simulink model "equivalent"  (R2018a)
settings: Solver=VariableStepAuto  StartTime=0.0  StopTime=10.0  RelTol=1e-3
undefined symbols (not defined in the file): DiscIntNeverNeededParam, sigbuilder_block
libraries: simulink x479
(part 2 of 10)

== system equivalent/cfblk286 ==
  cfblk1 : Inport
  Action Port : ActionPort  ActionType=else
  cfblk11 : Subsystem  TreatAsAtomicUnit=on
  cfblk12 : Subsystem  TreatAsAtomicUnit=on
  cfblk13 : Delay
  cfblk14 : Delay
  cfblk15 : Delay
  cfblk3 : DiscreteFir
  cfblk4 : simulink/Discrete/Transfer Fcn Real Zero  ZeroZ=0.75  ICPrevInput=0.0  DoSatur=off
      settings: SourceProductName=Simulink  SourceProductBaseCode=SL
  cfblk5 : DiscreteZeroPole  Poles=[0 0.5]  Gain=1  SampleTime=-1
  cfblk6 : simulink/Discrete/Difference  ICPrevInput=0.0  OutMin=[]  OutMax=[]  OutDataTypeStr=Inherit: Inherit via back propagation  OutDataType=fixdt(1, 16)  OutScaling=2^-10  DoSatur=off
  cfblk7 : Delay  ShowEnablePort=on
      settings: InputPortMap=u0,e6
  cfblk8 : DiscreteFir
  cfblk9 : If  SampleTime=1
  cyemi_{125,134..136,154..164} (15 alike) : DataTypeConversion  OutDataTypeStr=double
  cfblk2 : Outport
  cfblk10 : Outport  Port=2
  wires:
  cfblk6/1 -> cfblk2/1
  cfblk8/1 -> cyemi_155/1, cyemi_156/1
  cfblk5/1 -> cyemi_154/1, cyemi_160/1
  cfblk11/2(cfblk9) -> cfblk10/1
  cfblk12/1(cfblk2) -> cyemi_125/1, cyemi_162/1, cyemi_163/1
  cfblk9/1 -> cfblk11/Action
  cfblk9/2 -> cfblk12/Action
  cyemi_125/1 -> cfblk11/1(cfblk1)
  cyemi_134/1 -> cfblk12/1(cfblk1)
  cfblk1/1 -> cyemi_134/1
  cyemi_135/1 -> cfblk12/2(cfblk16)
  cfblk13/1 -> cyemi_135/1
  cyemi_136/1 -> cfblk12/3(cfblk17)
  cfblk15/1 -> cyemi_136/1
  cyemi_154/1 -> cfblk13/1
  cyemi_155/1 -> cfblk14/1
  cyemi_156/1 -> cfblk15/1
  cyemi_157/1 -> cfblk3/1
  cfblk7/1 -> cyemi_157/1
  cyemi_158/1 -> cfblk4/1
  cfblk11/1(cfblk2) -> cyemi_158/1
  cyemi_159/1 -> cfblk5/1
  cfblk3/1 -> cyemi_159/1
  cyemi_160/1 -> cfblk6/1
  cyemi_161/1 -> cfblk7/1
  cfblk4/1 -> cyemi_161/1
  cyemi_162/1 -> cfblk7/2
  cyemi_163/1 -> cfblk8/1
  cyemi_164/1 -> cfblk9/1
  cfblk14/1 -> cyemi_164/1

== system equivalent/cfblk287 ==
  cfblk1 : Inport
  cfblk12 : Inport  Port=2
  Action Port : ActionPort  ActionType=then
  cfblk10 : DiscreteTransferFcn
  cfblk11 : If  SampleTime=1
  cfblk15 : Subsystem  TreatAsAtomicUnit=on
  cfblk16 : Subsystem  TreatAsAtomicUnit=on
  cfblk{9,17..19} (4 alike) : Delay
  cfblk3 : Delay  DelayLengthSource=Input port
      settings: InputPortMap=u0,p1
  cfblk4 : simulink/Discrete/Transfer Fcn First Order  PoleZ=0.95  ICPrevOutput=0.0  DoSatur=off
      settings: SourceProductName=Simulink
  cfblk5 : DiscreteIntegrator  SampleTime=-1  ICPrevOutput=DiscIntNeverNeededParam  ICPrevScaledInput=DiscIntNeverNeededParam
  cfblk6 : simulink/Discrete/Transfer Fcn Real Zero  ZeroZ=0.75  ICPrevInput=0.0  DoSatur=off
      settings: SourceProductName=Simulink  SourceProductBaseCode=SL
  cfblk7 : Delay  ShowEnablePort=on
      settings: InputPortMap=u0,e6
  cfblk8 : simulink/Discrete/Transfer Fcn Real Zero  ZeroZ=0.75  ICPrevInput=0.0  DoSatur=off
      settings: SourceProductName=Simulink  SourceProductBaseCode=SL
  cyemi_{167..169,179..180,190..201} (17 alike) : DataTypeConversion  OutDataTypeStr=double
  cfblk2 : Outport
  cfblk13 : Outport  Port=2
  cfblk14 : Outport  Port=3
  wires:
  cfblk4/1 -> cfblk2/1
  cfblk7/1 -> cfblk14/1, cyemi_180/1
  cfblk15/3(cfblk12) -> cfblk13/1
  cfblk10/1 -> cyemi_179/1, cyemi_194/1
  cfblk11/1 -> cfblk15/Action
  cfblk11/2 -> cfblk16/Action
  cyemi_167/1 -> cfblk10/1
  cfblk1/1 -> cyemi_167/1
  cyemi_168/1 -> cfblk11/1
  cfblk19/1 -> cyemi_168/1
  cyemi_169/1 -> cfblk15/1(cfblk1)
  cfblk17/1 -> cyemi_169/1
  cyemi_179/1 -> cfblk16/1(cfblk1)
  cyemi_180/1 -> cfblk16/2(cfblk12)
  cyemi_190/1 -> cfblk17/1
  cfblk8/1 -> cyemi_190/1
  cyemi_191/1 -> cfblk18/1
  cfblk15/2(cfblk11) -> cyemi_191/1
  cyemi_192/1 -> cfblk19/1
  cfblk6/1 -> cyemi_192/1
  cyemi_193/1 -> cfblk3/1
  cfblk18/1 -> cyemi_193/1
  cyemi_194/1 -> cfblk3/2
  cyemi_195/1 -> cfblk4/1
  cfblk15/1(cfblk2) -> cyemi_195/1
  cyemi_196/1 -> cfblk5/1
  cfblk12/1 -> cyemi_196/1
  cyemi_197/1 -> cfblk6/1
  cfblk9/1 -> cyemi_197/1
  cyemi_198/1 -> cfblk7/1
  cfblk3/1 -> cyemi_198/1
  cyemi_199/1 -> cfblk7/2
  cfblk5/1 -> cyemi_199/1
  cyemi_200/1 -> cfblk8/1
  cfblk16/1(cfblk2) -> cyemi_200/1
  cyemi_201/1 -> cfblk9/1
  cfblk16/2(cfblk13) -> cyemi_201/1

== system equivalent/cfblk288 ==
  cfblk1 : Inport
  cfblk7 : Inport  Port=2
  Action Port : ActionPort  ActionType=else
  cfblk3 : DiscreteStateSpace  SampleTime=-1
  cfblk4 : simulink/Discrete/Transfer Fcn Real Zero  ZeroZ=0.75  ICPrevInput=0.0  DoSatur=off
      settings: SourceProductName=Simulink  SourceProductBaseCode=SL
  cfblk5 : simulink/Continuous/PID Controller (2DOF)  Controller=PID  TimeDomain=Discrete-time  SampleTime=-1  IntegratorMethod=Forward Euler  FilterMethod=Forward Euler  Form=Parallel  UseFilter=on  ControllerParametersSource=internal  P=1  I=1  D=0  N=100  b=1  c=1  InitialConditionSource=internal  InitialConditionForIntegrator=0  InitialConditionForFilter=0  ExternalReset=none  LimitOutput=off  UpperSaturationLimit=inf  LowerSaturationLimit=-inf  LinearizeAsGain=off  AntiWindupMode=none  Kb=1  TrackingMode=off  Kt=1  PParamMin=[]  PParamMax=[]  IParamMin=[]  IParamMax=[]  DParamMin=[]  DParamMax=[]  NParamMin=[]  NParamMax=[]  bParamMin=[]  bParamMax=[]  cParamMin=[]  cParamMax=[]  KbParamMin=[]  KbParamMax=[]  KtParamMin=[]  KtParamMax=[]  POutMin=[]  POutMax=[]  IOutMin=[]  IOutMax=[]  DOutMin=[]  DOutMax=[]  NOutMin=[]  NOutMax=[]  bOutMin=[]  bOutMax=[]  cOutMin=[]  cOutMax=[]  KbOutMin=[]  KbOutMax=[]  KtOutMin=[]  KtOutMax=[]  IntegratorOutMin=[]  IntegratorOutMax=[]  FilterOutMin=[]  FilterOutMax=[]  SumOutMin=[]  SumOutMax=[]  Sum1OutMin=[]  Sum1OutMax=[]  Sum2OutMin=[]  Sum2OutMax=[]  Sum3OutMin=[]  Sum3OutMax=[]  SumI1OutMin=[]  SumI1OutMax=[]  SumI2OutMin=[]  SumI2OutMax=[]  SumI3OutMin=[]  SumI3OutMax=[]  SumDOutMin=[]  SumDOutMax=[]  SaturationOutMin=[]  SaturationOutMax=[]  IntegratorContinuousStateAttributes=''  IntegratorStateMustResolveToSignalObject=off  IntegratorRTWStateStorageClass=Auto  FilterContinuousStateAttributes=''  FilterStateMustResolveToSignalObject=off  FilterRTWStateStorageClass=Auto  DifferentiatorICPrevScaledInput=0  DifferentiatorOutMin=[]  DifferentiatorOutMax=[]  FilterDiffOutCoefMin=[]  FilterDiffOutCoefMax=[]  SumDenOutMin=[]  SumDenOutMax=[]  SumNumOutMin=[]  SumNumOutMax=[]  ReciprocalOutMin=[]  ReciprocalOutMax=[]  DivideOutMin=[]  DivideOutMax=[]  TunerSelectOption=Transfer Function Based (PID Tuner App)
  cfblk6 : Delay  ShowEnablePort=on
      settings: InputPortMap=u0,e6
  cyemi_{204..209} (6 alike) : DataTypeConversion  OutDataTypeStr=double
  cfblk2 : Outport
  cfblk8 : Outport  Port=2
  cfblk9 : Outport  Port=3
  wires:
  cfblk6/1 -> cfblk2/1
  cfblk3/1 -> cfblk8/1, cyemi_206/1
  cfblk7/1 -> cfblk9/1, cyemi_205/1, cyemi_207/1
  cyemi_204/1 -> cfblk3/1
  cfblk1/1 -> cyemi_204/1
  cyemi_205/1 -> cfblk4/1
  cyemi_206/1 -> cfblk5/1
  cyemi_207/1 -> cfblk5/2
  cyemi_208/1 -> cfblk6/1
  cfblk5/1 -> cyemi_208/1
  cyemi_209/1 -> cfblk6/2
  cfblk4/1 -> cyemi_209/1

== system equivalent/cfblk289 ==
  cfblk1 : Inport
  cfblk6 : Inport  Port=2
  Action Port : ActionPort  ActionType=then
  cfblk3 : DiscreteZeroPole  Poles=[0 0.5]  Gain=1  SampleTime=-1
  cfblk4 : DiscreteFilter
  cfblk5 : DiscreteStateSpace  SampleTime=-1
  cyemi_212 : DataTypeConversion  OutDataTypeStr=double
  cyemi_213 : DataTypeConversion  OutDataTypeStr=double
  cyemi_214 : DataTypeConversion  OutDataTypeStr=double
  cfblk2 : Outport
  cfblk7 : Outport  Port=2
  wires:
  cfblk4/1 -> cfblk2/1
  cfblk1/1 -> cfblk7/1
  cyemi_212/1 -> cfblk3/1
  cfblk5/1 -> cyemi_212/1
  cyemi_213/1 -> cfblk4/1
  cfblk3/1 -> cyemi_213/1
  cyemi_214/1 -> cfblk5/1
  cfblk6/1 -> cyemi_214/1

== system equivalent/cfblk290 ==
  cfblk1 : Inport
  cfblk9 : Inport  Port=2
  cfblk10 : Inport  Port=3
  Action Port : ActionPort  ActionType=else
  cfblk12 : Delay
  cfblk3 : DiscreteZeroPole  Poles=[0 0.5]  Gain=1  SampleTime=-1
  cfblk4 : simulink/Discrete/Tapped Delay  vinit=0.0  samptime=-1  NumDelays=1  DelayOrder=Oldest  includeCurrent=off
  cfblk5 : Delay  ShowEnablePort=on
      settings: InputPortMap=u0,e6
  cfblk6 : simulink/Continuous/PID Controller (2DOF)  Controller=PID  TimeDomain=Discrete-time  SampleTime=-1  IntegratorMethod=Forward Euler  FilterMethod=Forward Euler  Form=Parallel  UseFilter=on  ControllerParametersSource=internal  P=1  I=1  D=0  N=100  b=1  c=1  InitialConditionSource=internal  InitialConditionForIntegrator=0  InitialConditionForFilter=0  ExternalReset=none  LimitOutput=off  UpperSaturationLimit=inf  LowerSaturationLimit=-inf  LinearizeAsGain=off  AntiWindupMode=none  Kb=1  TrackingMode=off  Kt=1  PParamMin=[]  PParamMax=[]  IParamMin=[]  IParamMax=[]  DParamMin=[]  DParamMax=[]  NParamMin=[]  NParamMax=[]  bParamMin=[]  bParamMax=[]  cParamMin=[]  cParamMax=[]  KbParamMin=[]  KbParamMax=[]  KtParamMin=[]  KtParamMax=[]  POutMin=[]  POutMax=[]  IOutMin=[]  IOutMax=[]  DOutMin=[]  DOutMax=[]  NOutMin=[]  NOutMax=[]  bOutMin=[]  bOutMax=[]  cOutMin=[]  cOutMax=[]  KbOutMin=[]  KbOutMax=[]  KtOutMin=[]  KtOutMax=[]  IntegratorOutMin=[]  IntegratorOutMax=[]  FilterOutMin=[]  FilterOutMax=[]  SumOutMin=[]  SumOutMax=[]  Sum1OutMin=[]  Sum1OutMax=[]  Sum2OutMin=[]  Sum2OutMax=[]  Sum3OutMin=[]  Sum3OutMax=[]  SumI1OutMin=[]  SumI1OutMax=[]  SumI2OutMin=[]  SumI2OutMax=[]  SumI3OutMin=[]  SumI3OutMax=[]  SumDOutMin=[]  SumDOutMax=[]  SaturationOutMin=[]  SaturationOutMax=[]  IntegratorContinuousStateAttributes=''  IntegratorStateMustResolveToSignalObject=off  IntegratorRTWStateStorageClass=Auto  FilterContinuousStateAttributes=''  FilterStateMustResolveToSignalObject=off  FilterRTWStateStorageClass=Auto  DifferentiatorICPrevScaledInput=0  DifferentiatorOutMin=[]  DifferentiatorOutMax=[]  FilterDiffOutCoefMin=[]  FilterDiffOutCoefMax=[]  SumDenOutMin=[]  SumDenOutMax=[]  SumNumOutMin=[]  SumNumOutMax=[]  ReciprocalOutMin=[]  ReciprocalOutMax=[]  DivideOutMin=[]  DivideOutMax=[]  TunerSelectOption=Transfer Function Based (PID Tuner App)
  cfblk7 : simulink/Discrete/Difference  ICPrevInput=0.0  OutMin=[]  OutMax=[]  OutDataTypeStr=Inherit: Inherit via back propagation  OutDataType=fixdt(1, 16)  OutScaling=2^-10  DoSatur=off
  cfblk8 : DiscreteIntegrator  SampleTime=-1  ICPrevOutput=DiscIntNeverNeededParam  ICPrevScaledInput=DiscIntNeverNeededParam
  cyemi_{219..227} (9 alike) : DataTypeConversion  OutDataTypeStr=double
  cfblk2 : Outport
  cfblk11 : Outport  Port=2
  wires:
  cfblk10/1 -> cyemi_223/1, cyemi_225/1
  cfblk6/1 -> cfblk11/1
  cfblk9/1 -> cfblk2/1
  cyemi_219/1 -> cfblk12/1
  cfblk5/1 -> cyemi_219/1
  cyemi_220/1 -> cfblk3/1
  cfblk12/1 -> cyemi_220/1
  cyemi_221/1 -> cfblk4/1
  cfblk8/1 -> cyemi_221/1
  cyemi_222/1 -> cfblk5/1
  cfblk3/1 -> cyemi_222/1
  cyemi_223/1 -> cfblk5/2
  cyemi_224/1 -> cfblk6/1
  cfblk7/1 -> cyemi_224/1
  cyemi_225/1 -> cfblk6/2
  cyemi_226/1 -> cfblk7/1
  cfblk4/1 -> cyemi_226/1
  cyemi_227/1 -> cfblk8/1
  cfblk1/1 -> cyemi_227/1

== system equivalent/cfblk291 ==
  cfblk1 : Inport
  cfblk7 : Inport  Port=2
  Action Port : ActionPort  ActionType=then
  cfblk3 : simulink/Discrete/Tapped Delay  vinit=0.0  samptime=-1  NumDelays=1  DelayOrder=Oldest  includeCurrent=off
  cfblk4 : simulink/Continuous/PID Controller  Controller=PID  TimeDomain=Discrete-time  SampleTime=-1  IntegratorMethod=Forward Euler  FilterMethod=Forward Euler  Form=Parallel  UseFilter=on  ControllerParametersSource=internal  P=1  I=1  D=0  N=100  InitialConditionSource=internal  InitialConditionForIntegrator=0  InitialConditionForFilter=0  ExternalReset=none  LimitOutput=off  UpperSaturationLimit=inf  LowerSaturationLimit=-inf  LinearizeAsGain=off  AntiWindupMode=none  Kb=1  TrackingMode=off  Kt=1  PParamMin=[]  PParamMax=[]  IParamMin=[]  IParamMax=[]  DParamMin=[]  DParamMax=[]  NParamMin=[]  NParamMax=[]  KbParamMin=[]  KbParamMax=[]  KtParamMin=[]  KtParamMax=[]  POutMin=[]  POutMax=[]  IOutMin=[]  IOutMax=[]  DOutMin=[]  DOutMax=[]  NOutMin=[]  NOutMax=[]  KbOutMin=[]  KbOutMax=[]  KtOutMin=[]  KtOutMax=[]  IntegratorOutMin=[]  IntegratorOutMax=[]  FilterOutMin=[]  FilterOutMax=[]  SumOutMin=[]  SumOutMax=[]  SumI1OutMin=[]  SumI1OutMax=[]  SumI2OutMin=[]  SumI2OutMax=[]  SumI3OutMin=[]  SumI3OutMax=[]  SumDOutMin=[]  SumDOutMax=[]  SaturationOutMin=[]  SaturationOutMax=[]  IntegratorContinuousStateAttributes=''  IntegratorStateMustResolveToSignalObject=off  IntegratorRTWStateStorageClass=Auto  FilterContinuousStateAttributes=''  FilterStateMustResolveToSignalObject=off  FilterRTWStateStorageClass=Auto  DifferentiatorICPrevScaledInput=0  DifferentiatorOutMin=[]  DifferentiatorOutMax=[]  FilterDiffOutCoefMin=[]  FilterDiffOutCoefMax=[]  SumDenOutMin=[]  SumDenOutMax=[]  SumNumOutMin=[]  SumNumOutMax=[]  ReciprocalOutMin=[]  ReciprocalOutMax=[]  DivideOutMin=[]  DivideOutMax=[]  TunerSelectOption=Transfer Function Based (PID Tuner App)
  cfblk5 : DiscreteFilter
  cfblk6 : UnitDelay  SampleTime=-1
  cyemi_{230..233} (4 alike) : DataTypeConversion  OutDataTypeStr=double
  cfblk2 : Outport
  cfblk8 : Outport  Port=2
  cfblk9 : Outport  Port=3
  wires:
  cfblk5/1 -> cfblk2/1
  cfblk4/1 -> cfblk8/1
  cfblk3/1 -> cfblk9/1
  cfblk1/1 -> cyemi_232/1, cyemi_233/1
  cyemi_230/1 -> cfblk3/1
  cfblk7/1 -> cyemi_230/1
  cyemi_231/1 -> cfblk4/1
  cfblk6/1 -> cyemi_231/1
  cyemi_232/1 -> cfblk5/1
  cyemi_233/1 -> cfblk6/1

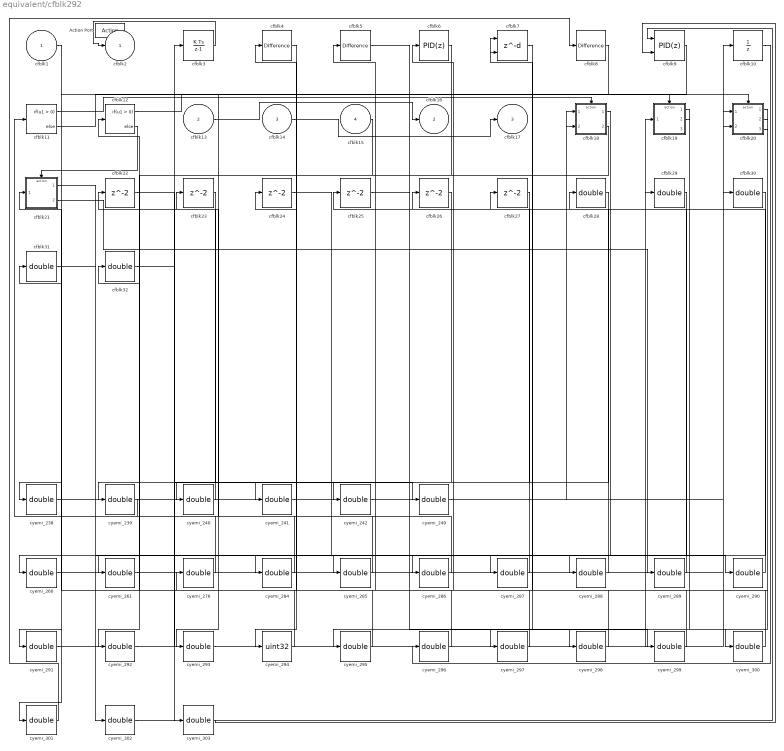
== system equivalent/cfblk292 ==
  cfblk1 : Inport
  cfblk13 : Inport  Port=2
  cfblk14 : Inport  Port=3
  cfblk15 : Inport  Port=4
  Action Port : ActionPort  ActionType=else
  cfblk10 : UnitDelay  SampleTime=-1
  cfblk11 : If  SampleTime=1
  cfblk12 : If  SampleTime=1
  cfblk18 : Subsystem  TreatAsAtomicUnit=on
  cfblk19 : Subsystem  TreatAsAtomicUnit=on
  cfblk20 : Subsystem  TreatAsAtomicUnit=on
  cfblk21 : Subsystem  TreatAsAtomicUnit=on
  cfblk{22..27} (6 alike) : Delay
  cfblk{28..32} (5 alike) : DataTypeConversion  OutDataTypeStr=double
  cfblk3 : DiscreteIntegrator  SampleTime=-1  ICPrevOutput=DiscIntNeverNeededParam  ICPrevScaledInput=DiscIntNeverNeededParam
  cfblk4 : simulink/Discrete/Difference  ICPrevInput=0.0  OutMin=[]  OutMax=[]  OutDataTypeStr=Inherit: Inherit via back propagation  OutDataType=fixdt(1, 16)  OutScaling=2^-10  DoSatur=off
  cfblk5 : simulink/Discrete/Difference  ICPrevInput=0.0  OutMin=[]  OutMax=[]  OutDataTypeStr=Inherit: Inherit via back propagation  OutDataType=fixdt(1, 16)  OutScaling=2^-10  DoSatur=off
  cfblk6 : simulink/Continuous/PID Controller  Controller=PID  TimeDomain=Discrete-time  SampleTime=-1  IntegratorMethod=Forward Euler  FilterMethod=Forward Euler  Form=Parallel  UseFilter=on  ControllerParametersSource=internal  P=1  I=1  D=0  N=100  InitialConditionSource=internal  InitialConditionForIntegrator=0  InitialConditionForFilter=0  ExternalReset=none  LimitOutput=off  UpperSaturationLimit=inf  LowerSaturationLimit=-inf  LinearizeAsGain=off  AntiWindupMode=none  Kb=1  TrackingMode=off  Kt=1  PParamMin=[]  PParamMax=[]  IParamMin=[]  IParamMax=[]  DParamMin=[]  DParamMax=[]  NParamMin=[]  NParamMax=[]  KbParamMin=[]  KbParamMax=[]  KtParamMin=[]  KtParamMax=[]  POutMin=[]  POutMax=[]  IOutMin=[]  IOutMax=[]  DOutMin=[]  DOutMax=[]  NOutMin=[]  NOutMax=[]  KbOutMin=[]  KbOutMax=[]  KtOutMin=[]  KtOutMax=[]  IntegratorOutMin=[]  IntegratorOutMax=[]  FilterOutMin=[]  FilterOutMax=[]  SumOutMin=[]  SumOutMax=[]  SumI1OutMin=[]  SumI1OutMax=[]  SumI2OutMin=[]  SumI2OutMax=[]  SumI3OutMin=[]  SumI3OutMax=[]  SumDOutMin=[]  SumDOutMax=[]  SaturationOutMin=[]  SaturationOutMax=[]  IntegratorContinuousStateAttributes=''  IntegratorStateMustResolveToSignalObject=off  IntegratorRTWStateStorageClass=Auto  FilterContinuousStateAttributes=''  FilterStateMustResolveToSignalObject=off  FilterRTWStateStorageClass=Auto  DifferentiatorICPrevScaledInput=0  DifferentiatorOutMin=[]  DifferentiatorOutMax=[]  FilterDiffOutCoefMin=[]  FilterDiffOutCoefMax=[]  SumDenOutMin=[]  SumDenOutMax=[]  SumNumOutMin=[]  SumNumOutMax=[]  ReciprocalOutMin=[]  ReciprocalOutMax=[]  DivideOutMin=[]  DivideOutMax=[]  TunerSelectOption=Transfer Function Based (PID Tuner App)
  cfblk7 : Delay  DelayLengthSource=Input port
      settings: InputPortMap=u0,p1
  cfblk8 : simulink/Discrete/Difference  ICPrevInput=0.0  OutMin=[]  OutMax=[]  OutDataTypeStr=Inherit: Inherit via back propagation  OutDataType=fixdt(1, 16)  OutScaling=2^-10  DoSatur=off
  cfblk9 : simulink/Continuous/PID Controller (2DOF)  Controller=PID  TimeDomain=Discrete-time  SampleTime=-1  IntegratorMethod=Forward Euler  FilterMethod=Forward Euler  Form=Parallel  UseFilter=on  ControllerParametersSource=internal  P=1  I=1  D=0  N=100  b=1  c=1  InitialConditionSource=internal  InitialConditionForIntegrator=0  InitialConditionForFilter=0  ExternalReset=none  LimitOutput=off  UpperSaturationLimit=inf  LowerSaturationLimit=-inf  LinearizeAsGain=off  AntiWindupMode=none  Kb=1  TrackingMode=off  Kt=1  PParamMin=[]  PParamMax=[]  IParamMin=[]  IParamMax=[]  DParamMin=[]  DParamMax=[]  NParamMin=[]  NParamMax=[]  bParamMin=[]  bParamMax=[]  cParamMin=[]  cParamMax=[]  KbParamMin=[]  KbParamMax=[]  KtParamMin=[]  KtParamMax=[]  POutMin=[]  POutMax=[]  IOutMin=[]  IOutMax=[]  DOutMin=[]  DOutMax=[]  NOutMin=[]  NOutMax=[]  bOutMin=[]  bOutMax=[]  cOutMin=[]  cOutMax=[]  KbOutMin=[]  KbOutMax=[]  KtOutMin=[]  KtOutMax=[]  IntegratorOutMin=[]  IntegratorOutMax=[]  FilterOutMin=[]  FilterOutMax=[]  SumOutMin=[]  SumOutMax=[]  Sum1OutMin=[]  Sum1OutMax=[]  Sum2OutMin=[]  Sum2OutMax=[]  Sum3OutMin=[]  Sum3OutMax=[]  SumI1OutMin=[]  SumI1OutMax=[]  SumI2OutMin=[]  SumI2OutMax=[]  SumI3OutMin=[]  SumI3OutMax=[]  SumDOutMin=[]  SumDOutMax=[]  SaturationOutMin=[]  SaturationOutMax=[]  IntegratorContinuousStateAttributes=''  IntegratorStateMustResolveToSignalObject=off  IntegratorRTWStateStorageClass=Auto  FilterContinuousStateAttributes=''  FilterStateMustResolveToSignalObject=off  FilterRTWStateStorageClass=Auto  DifferentiatorICPrevScaledInput=0  DifferentiatorOutMin=[]  DifferentiatorOutMax=[]  FilterDiffOutCoefMin=[]  FilterDiffOutCoefMax=[]  SumDenOutMin=[]  SumDenOutMax=[]  SumNumOutMin=[]  SumNumOutMax=[]  ReciprocalOutMin=[]  ReciprocalOutMax=[]  DivideOutMin=[]  DivideOutMax=[]  TunerSelectOption=Transfer Function Based (PID Tuner App)
  cyemi_{238..242,249,260..261,276,284..293,295..303} (28 alike) : DataTypeConversion  OutDataTypeStr=double
  cyemi_294 : DataTypeConversion  OutDataTypeStr=uint32
  cfblk2 : Outport
  cfblk16 : Outport  Port=2
  cfblk17 : Outport  Port=3
  wires:
  cfblk14/1 -> cfblk17/1
  cfblk3/1 -> cfblk2/1
  cfblk13/1 -> cfblk16/1
  cfblk11/1 -> cfblk18/Action
  cfblk11/2 -> cfblk19/Action
  cfblk12/1 -> cfblk20/Action
  cfblk12/2 -> cfblk21/Action
  cyemi_238/1 -> cfblk10/1
  cfblk8/1 -> cyemi_238/1
  cyemi_239/1 -> cfblk11/1
  cfblk28/1 -> cyemi_239/1
  cyemi_240/1 -> cfblk12/1
  cfblk27/1 -> cyemi_240/1
  cyemi_241/1 -> cfblk18/1(cfblk1)
  cfblk4/1 -> cyemi_241/1
  cyemi_242/1 -> cfblk18/2(cfblk9)
  cfblk26/1 -> cyemi_242/1
  cyemi_249/1 -> cfblk19/1(cfblk1)
  cfblk22/1 -> cyemi_249/1
  cyemi_260/1 -> cfblk20/1(cfblk1)
  cfblk18/1(cfblk2) -> cyemi_260/1
  cyemi_261/1 -> cfblk20/2(cfblk14)
  cfblk23/1 -> cyemi_261/1
  cyemi_276/1 -> cfblk21/1(cfblk1)
  cfblk20/3(cfblk16) -> cyemi_276/1
  cyemi_284/1 -> cfblk22/1
  cfblk6/1 -> cyemi_284/1
  cyemi_285/1 -> cfblk23/1
  cfblk19/1(cfblk2) -> cyemi_285/1
  cyemi_286/1 -> cfblk24/1
  cfblk29/1 -> cyemi_286/1
  cyemi_287/1 -> cfblk25/1
  cfblk5/1 -> cyemi_287/1
  cyemi_288/1 -> cfblk26/1
  cfblk21/1(cfblk2) -> cyemi_288/1
  cyemi_289/1 -> cfblk27/1
  cfblk21/2(cfblk8) -> cyemi_289/1
  cyemi_290/1 -> cfblk28/1
  cfblk24/1 -> cyemi_290/1
  cyemi_291/1 -> cfblk29/1
  cfblk30/1 -> cyemi_291/1
  cyemi_292/1 -> cfblk3/1
  cfblk18/2(cfblk10) -> cyemi_292/1
  cyemi_293/1 -> cfblk30/1
  cfblk9/1 -> cyemi_293/1
  cyemi_294/1 -> cfblk31/1
  cfblk15/1 -> cyemi_294/1
  cyemi_295/1 -> cfblk32/1
  cfblk19/2(cfblk9) -> cyemi_295/1
  cyemi_296/1 -> cfblk4/1
  cfblk10/1 -> cyemi_296/1
  cyemi_297/1 -> cfblk5/1
  cfblk7/1 -> cyemi_297/1
  cyemi_298/1 -> cfblk6/1
  cfblk20/1(cfblk2) -> cyemi_298/1
  cyemi_299/1 -> cfblk7/1
  cfblk25/1 -> cyemi_299/1
  cyemi_300/1 -> cfblk7/2
  cfblk20/2(cfblk15) -> cyemi_300/1
  cyemi_301/1 -> cfblk8/1
  cfblk1/1 -> cyemi_301/1
  cyemi_302/1 -> cfblk9/1
  cfblk31/1 -> cyemi_302/1
  cyemi_303/1 -> cfblk9/2
  cfblk32/1 -> cyemi_303/1

== system equivalent/cfblk293 ==
  cfblk1 : Inport
  cfblk10 : Inport  Port=2
  cfblk11 : Inport  Port=3
  Action Port : ActionPort  ActionType=then
  cfblk13 : Subsystem  TreatAsAtomicUnit=on
  cfblk14 : Subsystem  TreatAsAtomicUnit=on
  cfblk15 : Delay
  cfblk16 : Delay
  cfblk3 : DiscreteIntegrator  SampleTime=-1  ICPrevOutput=DiscIntNeverNeededParam  ICPrevScaledInput=DiscIntNeverNeededParam
  cfblk4 : DiscreteStateSpace  SampleTime=-1
  cfblk5 : DiscreteTransferFcn
  cfblk6 : UnitDelay  SampleTime=-1
  cfblk7 : simulink/Discrete/Difference  ICPrevInput=0.0  OutMin=[]  OutMax=[]  OutDataTypeStr=Inherit: Inherit via back propagation  OutDataType=fixdt(1, 16)  OutScaling=2^-10  DoSatur=off
  cfblk8 : simulink/Continuous/PID Controller  Controller=PID  TimeDomain=Discrete-time  SampleTime=-1  IntegratorMethod=Forward Euler  FilterMethod=Forward Euler  Form=Parallel  UseFilter=on  ControllerParametersSource=internal  P=1  I=1  D=0  N=100  InitialConditionSource=internal  InitialConditionForIntegrator=0  InitialConditionForFilter=0  ExternalReset=none  LimitOutput=off  UpperSaturationLimit=inf  LowerSaturationLimit=-inf  LinearizeAsGain=off  AntiWindupMode=none  Kb=1  TrackingMode=off  Kt=1  PParamMin=[]  PParamMax=[]  IParamMin=[]  IParamMax=[]  DParamMin=[]  DParamMax=[]  NParamMin=[]  NParamMax=[]  KbParamMin=[]  KbParamMax=[]  KtParamMin=[]  KtParamMax=[]  POutMin=[]  POutMax=[]  IOutMin=[]  IOutMax=[]  DOutMin=[]  DOutMax=[]  NOutMin=[]  NOutMax=[]  KbOutMin=[]  KbOutMax=[]  KtOutMin=[]  KtOutMax=[]  IntegratorOutMin=[]  IntegratorOutMax=[]  FilterOutMin=[]  FilterOutMax=[]  SumOutMin=[]  SumOutMax=[]  SumI1OutMin=[]  SumI1OutMax=[]  SumI2OutMin=[]  SumI2OutMax=[]  SumI3OutMin=[]  SumI3OutMax=[]  SumDOutMin=[]  SumDOutMax=[]  SaturationOutMin=[]  SaturationOutMax=[]  IntegratorContinuousStateAttributes=''  IntegratorStateMustResolveToSignalObject=off  IntegratorRTWStateStorageClass=Auto  FilterContinuousStateAttributes=''  FilterStateMustResolveToSignalObject=off  FilterRTWStateStorageClass=Auto  DifferentiatorICPrevScaledInput=0  DifferentiatorOutMin=[]  DifferentiatorOutMax=[]  FilterDiffOutCoefMin=[]  FilterDiffOutCoefMax=[]  SumDenOutMin=[]  SumDenOutMax=[]  SumNumOutMin=[]  SumNumOutMax=[]  ReciprocalOutMin=[]  ReciprocalOutMax=[]  DivideOutMin=[]  DivideOutMax=[]  TunerSelectOption=Transfer Function Based (PID Tuner App)
  cfblk9 : If  SampleTime=1
  cyemi_{307..308,326..327,340..348} (13 alike) : DataTypeConversion  OutDataTypeStr=double
  cfblk2 : Outport
  cfblk12 : Outport  Port=2
  wires:
  cfblk8/1 -> cfblk12/1
  cfblk14/2(cfblk12) -> cfblk2/1
  cfblk9/1 -> cfblk13/Action
  cfblk9/2 -> cfblk14/Action
  cyemi_307/1 -> cfblk13/1(cfblk1)
  cfblk1/1 -> cyemi_307/1
  cyemi_308/1 -> cfblk13/2(cfblk12)
  cfblk16/1 -> cyemi_308/1
  cyemi_326/1 -> cfblk14/1(cfblk1)
  cfblk15/1 -> cyemi_326/1
  cyemi_327/1 -> cfblk14/2(cfblk11)
  cfblk7/1 -> cyemi_327/1
  cyemi_340/1 -> cfblk15/1
  cfblk4/1 -> cyemi_340/1
  cyemi_341/1 -> cfblk16/1
  cfblk14/3(cfblk13) -> cyemi_341/1
  cyemi_342/1 -> cfblk3/1
  cfblk13/1(cfblk2) -> cyemi_342/1
  cyemi_343/1 -> cfblk4/1
  cfblk3/1 -> cyemi_343/1
  cyemi_344/1 -> cfblk5/1
  cfblk11/1 -> cyemi_344/1
  cyemi_345/1 -> cfblk6/1
  cfblk5/1 -> cyemi_345/1
  cyemi_346/1 -> cfblk7/1
  cfblk10/1 -> cyemi_346/1
  cyemi_347/1 -> cfblk8/1
  cfblk14/1(cfblk2) -> cyemi_347/1
  cyemi_348/1 -> cfblk9/1
  cfblk6/1 -> cyemi_348/1

== system equivalent/cfblk294 ==
  cfblk1 : Inport
  cfblk12 : Inport  Port=2
  cfblk13 : Inport  Port=3
  Action Port : ActionPort  ActionType=else
  cfblk10 : DiscreteIntegrator  SampleTime=-1  ICPrevOutput=DiscIntNeverNeededParam  ICPrevScaledInput=DiscIntNeverNeededParam
  cfblk11 : DiscreteZeroPole  Poles=[0 0.5]  Gain=1  SampleTime=-1
  cfblk3 : DiscreteFilter
  cfblk4 : DiscreteZeroPole  Poles=[0 0.5]  Gain=1  SampleTime=-1
  cfblk5 : simulink/Discrete/Transfer Fcn Real Zero  ZeroZ=0.75  ICPrevInput=0.0  DoSatur=off
      settings: SourceProductName=Simulink  SourceProductBaseCode=SL
  cfblk6 : DiscreteFilter
  cfblk7 : simulink/Discrete/Transfer Fcn Lead or Lag  PoleZ=0.95  ZeroZ=0.75  ICPrevOutput=0.0  ICPrevInput=0.0  DoSatur=off
      settings: SourceProductName=Simulink  SourceProductBaseCode=SL
  cfblk8 : simulink/Discrete/Tapped Delay  vinit=0.0  samptime=-1  NumDelays=1  DelayOrder=Oldest  includeCurrent=off
  cfblk9 : DiscreteIntegrator  SampleTime=-1  ICPrevOutput=DiscIntNeverNeededParam  ICPrevScaledInput=DiscIntNeverNeededParam
  cyemi_{352..360} (9 alike) : DataTypeConversion  OutDataTypeStr=double
  cfblk2 : Outport
  cfblk14 : Outport  Port=2
  wires:
  cfblk5/1 -> cfblk14/1
  cfblk12/1 -> cfblk2/1
  cyemi_352/1 -> cfblk10/1
  cfblk3/1 -> cyemi_352/1
  cyemi_353/1 -> cfblk11/1
  cfblk7/1 -> cyemi_353/1
  cyemi_354/1 -> cfblk3/1
  cfblk9/1 -> cyemi_354/1
  cyemi_355/1 -> cfblk4/1
  cfblk13/1 -> cyemi_355/1
  cyemi_356/1 -> cfblk5/1
  cfblk10/1 -> cyemi_356/1
  cyemi_357/1 -> cfblk6/1
  cfblk11/1 -> cyemi_357/1
  cyemi_358/1 -> cfblk7/1
  cfblk8/1 -> cyemi_358/1
  cyemi_359/1 -> cfblk8/1
  cfblk4/1 -> cyemi_359/1
  cyemi_360/1 -> cfblk9/1
  cfblk6/1 -> cyemi_360/1

== system equivalent/cfblk295 ==
  cfblk1 : Inport
  cfblk10 : Inport  Port=2
  Action Port : ActionPort  ActionType=then
  cfblk12 : Delay
  cfblk3 : simulink/Discrete/Transfer Fcn Real Zero  ZeroZ=0.75  ICPrevInput=0.0  DoSatur=off
      settings: SourceProductName=Simulink  SourceProductBaseCode=SL
  cfblk4 : Delay  ShowEnablePort=on
      settings: InputPortMap=u0,e6
  cfblk5 : Delay
  cfblk6 : Delay
  cfblk7 : DiscreteFilter
  cfblk8 : DiscreteIntegrator  SampleTime=-1  ICPrevOutput=DiscIntNeverNeededParam  ICPrevScaledInput=DiscIntNeverNeededParam
  cfblk9 : DiscreteFir
  cyemi_{363..371} (9 alike) : DataTypeConversion  OutDataTypeStr=double
  cfblk2 : Outport
  cfblk11 : Outport  Port=2
  wires:
  cfblk7/1 -> cyemi_370/1, cyemi_371/1
  cfblk8/1 -> cfblk2/1
  cfblk5/1 -> cfblk11/1
  cyemi_363/1 -> cfblk12/1
  cfblk4/1 -> cyemi_363/1
  cyemi_364/1 -> cfblk3/1
  cfblk12/1 -> cyemi_364/1
  cyemi_365/1 -> cfblk4/1
  cfblk10/1 -> cyemi_365/1
  cyemi_366/1 -> cfblk4/2
  cfblk6/1 -> cyemi_366/1
  cyemi_367/1 -> cfblk5/1
  cfblk1/1 -> cyemi_367/1
  cyemi_368/1 -> cfblk6/1
  cfblk9/1 -> cyemi_368/1
  cyemi_369/1 -> cfblk7/1
  cfblk3/1 -> cyemi_369/1
  cyemi_370/1 -> cfblk8/1
  cyemi_371/1 -> cfblk9/1

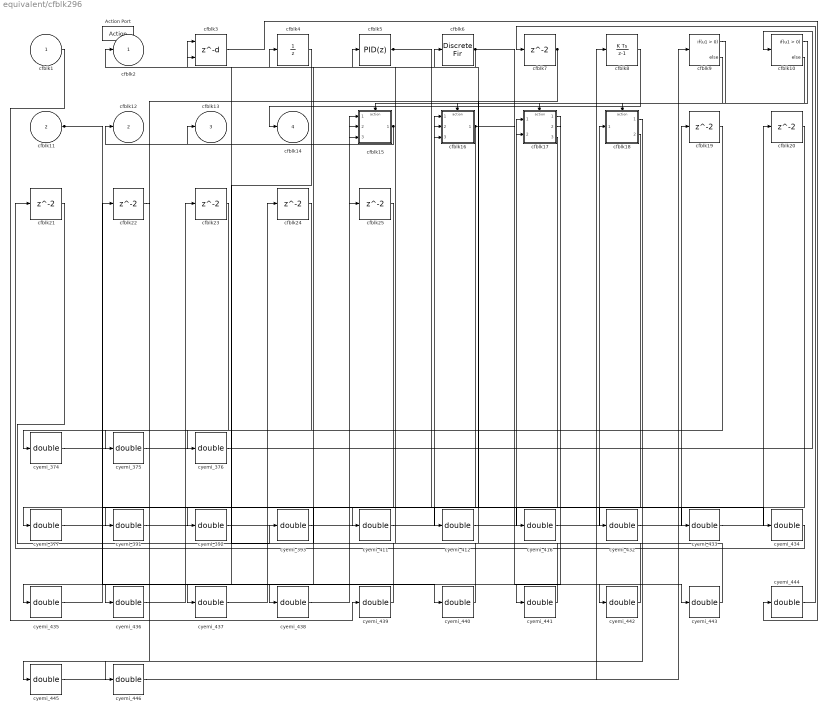
== system equivalent/cfblk296 ==
  cfblk1 : Inport
  cfblk11 : Inport  Port=2
  Action Port : ActionPort  ActionType=else
  cfblk10 : If  SampleTime=1
  cfblk15 : Subsystem  TreatAsAtomicUnit=on
  cfblk16 : Subsystem  TreatAsAtomicUnit=on
  cfblk17 : Subsystem  TreatAsAtomicUnit=on
  cfblk18 : Subsystem  TreatAsAtomicUnit=on
  cfblk{7,19..25} (8 alike) : Delay
  cfblk3 : Delay  DelayLengthSource=Input port
      settings: InputPortMap=u0,p1
  cfblk4 : UnitDelay  SampleTime=-1
  cfblk5 : simulink/Continuous/PID Controller  Controller=PID  TimeDomain=Discrete-time  SampleTime=-1  IntegratorMethod=Forward Euler  FilterMethod=Forward Euler  Form=Parallel  UseFilter=on  ControllerParametersSource=internal  P=1  I=1  D=0  N=100  InitialConditionSource=internal  InitialConditionForIntegrator=0  InitialConditionForFilter=0  ExternalReset=none  LimitOutput=off  UpperSaturationLimit=inf  LowerSaturationLimit=-inf  LinearizeAsGain=off  AntiWindupMode=none  Kb=1  TrackingMode=off  Kt=1  PParamMin=[]  PParamMax=[]  IParamMin=[]  IParamMax=[]  DParamMin=[]  DParamMax=[]  NParamMin=[]  NParamMax=[]  KbParamMin=[]  KbParamMax=[]  KtParamMin=[]  KtParamMax=[]  POutMin=[]  POutMax=[]  IOutMin=[]  IOutMax=[]  DOutMin=[]  DOutMax=[]  NOutMin=[]  NOutMax=[]  KbOutMin=[]  KbOutMax=[]  KtOutMin=[]  KtOutMax=[]  IntegratorOutMin=[]  IntegratorOutMax=[]  FilterOutMin=[]  FilterOutMax=[]  SumOutMin=[]  SumOutMax=[]  SumI1OutMin=[]  SumI1OutMax=[]  SumI2OutMin=[]  SumI2OutMax=[]  SumI3OutMin=[]  SumI3OutMax=[]  SumDOutMin=[]  SumDOutMax=[]  SaturationOutMin=[]  SaturationOutMax=[]  IntegratorContinuousStateAttributes=''  IntegratorStateMustResolveToSignalObject=off  IntegratorRTWStateStorageClass=Auto  FilterContinuousStateAttributes=''  FilterStateMustResolveToSignalObject=off  FilterRTWStateStorageClass=Auto  DifferentiatorICPrevScaledInput=0  DifferentiatorOutMin=[]  DifferentiatorOutMax=[]  FilterDiffOutCoefMin=[]  FilterDiffOutCoefMax=[]  SumDenOutMin=[]  SumDenOutMax=[]  SumNumOutMin=[]  SumNumOutMax=[]  ReciprocalOutMin=[]  ReciprocalOutMax=[]  DivideOutMin=[]  DivideOutMax=[]  TunerSelectOption=Transfer Function Based (PID Tuner App)
  cfblk6 : DiscreteFir
  cfblk8 : DiscreteIntegrator  SampleTime=-1  ICPrevOutput=DiscIntNeverNeededParam  ICPrevScaledInput=DiscIntNeverNeededParam
  cfblk9 : If  SampleTime=1
  cyemi_{374..377,391..393,411..412,416,432..446} (25 alike) : DataTypeConversion  OutDataTypeStr=double
  cfblk2 : Outport
  cfblk12 : Outport  Port=2
  cfblk13 : Outport  Port=3
  cfblk14 : Outport  Port=4
  wires:
  cfblk15/1(cfblk2) -> cfblk12/1, cfblk13/1
  cfblk7/1 -> cyemi_412/1, cyemi_446/1
  cfblk8/1 -> cfblk14/1
  cfblk11/1 -> cyemi_416/1, cyemi_440/1
  cfblk16/1(cfblk2) -> cyemi_411/1, cyemi_443/1
  cfblk5/1 -> cyemi_432/1, cyemi_433/1
  cfblk6/1 -> cfblk2/1, cyemi_434/1, cyemi_442/1
  cfblk9/1 -> cfblk15/Action
  cfblk9/2 -> cfblk16/Action
  cfblk10/1 -> cfblk17/Action
  cfblk10/2 -> cfblk18/Action
  cyemi_374/1 -> cfblk10/1
  cfblk23/1 -> cyemi_374/1
  cyemi_375/1 -> cfblk15/1(cfblk1)
  cfblk19/1 -> cyemi_375/1
  cyemi_376/1 -> cfblk15/2(cfblk12)
  cfblk24/1 -> cyemi_376/1
  cyemi_377/1 -> cfblk15/3(cfblk13)
  cfblk25/1 -> cyemi_377/1
  cyemi_391/1 -> cfblk16/1(cfblk1)
  cfblk22/1 -> cyemi_391/1
  cyemi_392/1 -> cfblk16/2(cfblk14)
  cfblk20/1 -> cyemi_392/1
  cyemi_393/1 -> cfblk16/3(cfblk15)
  cfblk21/1 -> cyemi_393/1
  cyemi_411/1 -> cfblk17/1(cfblk1)
  cyemi_412/1 -> cfblk17/2(cfblk6)
  cyemi_416/1 -> cfblk18/1(cfblk1)
  cyemi_432/1 -> cfblk19/1
  cyemi_433/1 -> cfblk20/1
  cyemi_434/1 -> cfblk21/1
  cyemi_435/1 -> cfblk22/1
  cfblk17/1(cfblk2) -> cyemi_435/1
  cyemi_436/1 -> cfblk23/1
  cfblk17/2(cfblk7) -> cyemi_436/1
  cyemi_437/1 -> cfblk24/1
  cfblk4/1 -> cyemi_437/1
  cyemi_438/1 -> cfblk25/1
  cfblk17/3(cfblk8) -> cyemi_438/1
  cyemi_439/1 -> cfblk3/1
  cfblk1/1 -> cyemi_439/1
  cyemi_440/1 -> cfblk3/2
  cyemi_441/1 -> cfblk4/1
  cfblk18/2(cfblk14) -> cyemi_441/1
  cyemi_442/1 -> cfblk5/1
  cyemi_443/1 -> cfblk6/1
  cyemi_444/1 -> cfblk7/1
  cfblk3/1 -> cyemi_444/1
  cyemi_445/1 -> cfblk8/1
  cfblk18/1(cfblk2) -> cyemi_445/1
  cyemi_446/1 -> cfblk9/1

== system equivalent/cfblk297 ==
  cfblk1 : Inport
  cfblk4 : Inport  Port=2
  Action Port : ActionPort  ActionType=then
  cfblk3 : DiscreteZeroPole  Poles=[0 0.5]  Gain=1  SampleTime=-1
  cyemi_449 : DataTypeConversion  OutDataTypeStr=double
  cfblk2 : Outport
  cfblk5 : Outport  Port=2
  cfblk6 : Outport  Port=3
  cfblk7 : Outport  Port=4
  wires:
  cfblk4/1 -> cfblk7/1, cfblk5/1
  cfblk1/1 -> cfblk2/1, cyemi_449/1
  cfblk3/1 -> cfblk6/1
  cyemi_449/1 -> cfblk3/1

== system equivalent/cfblk298 ==
  cfblk1 : Inport
  cfblk8 : Inport  Port=2
  Action Port : ActionPort  ActionType=else
  cfblk3 : simulink/Discrete/Tapped Delay  vinit=0.0  samptime=-1  NumDelays=1  DelayOrder=Oldest  includeCurrent=off
  cfblk4 : DiscreteZeroPole  Poles=[0 0.5]  Gain=1  SampleTime=-1
  cfblk5 : simulink/Discrete/Transfer Fcn Real Zero  ZeroZ=0.75  ICPrevInput=0.0  DoSatur=off
      settings: SourceProductName=Simulink  SourceProductBaseCode=SL
  cfblk6 : DiscreteIntegrator  SampleTime=-1  ICPrevOutput=DiscIntNeverNeededParam  ICPrevScaledInput=DiscIntNeverNeededParam
  cfblk7 : simulink/Discrete/Transfer Fcn Lead or Lag  PoleZ=0.95  ZeroZ=0.75  ICPrevOutput=0.0  ICPrevInput=0.0  DoSatur=off
      settings: SourceProductName=Simulink  SourceProductBaseCode=SL
  cyemi_{452..456} (5 alike) : DataTypeConversion  OutDataTypeStr=double
  cfblk2 : Outport
  cfblk9 : Outport  Port=2
  wires:
  cfblk6/1 -> cfblk9/1
  cfblk4/1 -> cfblk2/1
  cyemi_452/1 -> cfblk3/1
  cfblk1/1 -> cyemi_452/1
  cyemi_453/1 -> cfblk4/1
  cfblk7/1 -> cyemi_453/1
  cyemi_454/1 -> cfblk5/1
  cfblk8/1 -> cyemi_454/1
  cyemi_455/1 -> cfblk6/1
  cfblk5/1 -> cyemi_455/1
  cyemi_456/1 -> cfblk7/1
  cfblk3/1 -> cyemi_456/1

== system equivalent/cfblk299 ==
  cfblk1 : Inport
  cfblk12 : Inport  Port=2
  cfblk13 : Inport  Port=3
  Action Port : ActionPort  ActionType=then
  cfblk10 : Delay  ShowEnablePort=on
      settings: InputPortMap=u0,e6
  cfblk11 : If  SampleTime=1
  cfblk16 : Subsystem  TreatAsAtomicUnit=on
  cfblk17 : Subsystem  TreatAsAtomicUnit=on
  cfblk18 : Delay
  cfblk3 : DiscreteTransferFcn
  cfblk4 : simulink/Continuous/PID Controller  Controller=PID  TimeDomain=Discrete-time  SampleTime=-1  IntegratorMethod=Forward Euler  FilterMethod=Forward Euler  Form=Parallel  UseFilter=on  ControllerParametersSource=internal  P=1  I=1  D=0  N=100  InitialConditionSource=internal  InitialConditionForIntegrator=0  InitialConditionForFilter=0  ExternalReset=none  LimitOutput=off  UpperSaturationLimit=inf  LowerSaturationLimit=-inf  LinearizeAsGain=off  AntiWindupMode=none  Kb=1  TrackingMode=off  Kt=1  PParamMin=[]  PParamMax=[]  IParamMin=[]  IParamMax=[]  DParamMin=[]  DParamMax=[]  NParamMin=[]  NParamMax=[]  KbParamMin=[]  KbParamMax=[]  KtParamMin=[]  KtParamMax=[]  POutMin=[]  POutMax=[]  IOutMin=[]  IOutMax=[]  DOutMin=[]  DOutMax=[]  NOutMin=[]  NOutMax=[]  KbOutMin=[]  KbOutMax=[]  KtOutMin=[]  KtOutMax=[]  IntegratorOutMin=[]  IntegratorOutMax=[]  FilterOutMin=[]  FilterOutMax=[]  SumOutMin=[]  SumOutMax=[]  SumI1OutMin=[]  SumI1OutMax=[]  SumI2OutMin=[]  SumI2OutMax=[]  SumI3OutMin=[]  SumI3OutMax=[]  SumDOutMin=[]  SumDOutMax=[]  SaturationOutMin=[]  SaturationOutMax=[]  IntegratorContinuousStateAttributes=''  IntegratorStateMustResolveToSignalObject=off  IntegratorRTWStateStorageClass=Auto  FilterContinuousStateAttributes=''  FilterStateMustResolveToSignalObject=off  FilterRTWStateStorageClass=Auto  DifferentiatorICPrevScaledInput=0  DifferentiatorOutMin=[]  DifferentiatorOutMax=[]  FilterDiffOutCoefMin=[]  FilterDiffOutCoefMax=[]  SumDenOutMin=[]  SumDenOutMax=[]  SumNumOutMin=[]  SumNumOutMax=[]  ReciprocalOutMin=[]  ReciprocalOutMax=[]  DivideOutMin=[]  DivideOutMax=[]  TunerSelectOption=Transfer Function Based (PID Tuner App)
  cfblk5 : Delay  DelayLengthSource=Input port
      settings: InputPortMap=u0,p1
  cfblk6 : simulink/Discrete/Transfer Fcn Real Zero  ZeroZ=0.75  ICPrevInput=0.0  DoSatur=off
      settings: SourceProductName=Simulink  SourceProductBaseCode=SL
  cfblk7 : DiscreteFilter
  cfblk8 : simulink/Continuous/PID Controller  Controller=PID  TimeDomain=Discrete-time  SampleTime=-1  IntegratorMethod=Forward Euler  FilterMethod=Forward Euler  Form=Parallel  UseFilter=on  ControllerParametersSource=internal  P=1  I=1  D=0  N=100  InitialConditionSource=internal  InitialConditionForIntegrator=0  InitialConditionForFilter=0  ExternalReset=none  LimitOutput=off  UpperSaturationLimit=inf  LowerSaturationLimit=-inf  LinearizeAsGain=off  AntiWindupMode=none  Kb=1  TrackingMode=off  Kt=1  PParamMin=[]  PParamMax=[]  IParamMin=[]  IParamMax=[]  DParamMin=[]  DParamMax=[]  NParamMin=[]  NParamMax=[]  KbParamMin=[]  KbParamMax=[]  KtParamMin=[]  KtParamMax=[]  POutMin=[]  POutMax=[]  IOutMin=[]  IOutMax=[]  DOutMin=[]  DOutMax=[]  NOutMin=[]  NOutMax=[]  KbOutMin=[]  KbOutMax=[]  KtOutMin=[]  KtOutMax=[]  IntegratorOutMin=[]  IntegratorOutMax=[]  FilterOutMin=[]  FilterOutMax=[]  SumOutMin=[]  SumOutMax=[]  SumI1OutMin=[]  SumI1OutMax=[]  SumI2OutMin=[]  SumI2OutMax=[]  SumI3OutMin=[]  SumI3OutMax=[]  SumDOutMin=[]  SumDOutMax=[]  SaturationOutMin=[]  SaturationOutMax=[]  IntegratorContinuousStateAttributes=''  IntegratorStateMustResolveToSignalObject=off  IntegratorRTWStateStorageClass=Auto  FilterContinuousStateAttributes=''  FilterStateMustResolveToSignalObject=off  FilterRTWStateStorageClass=Auto  DifferentiatorICPrevScaledInput=0  DifferentiatorOutMin=[]  DifferentiatorOutMax=[]  FilterDiffOutCoefMin=[]  FilterDiffOutCoefMax=[]  SumDenOutMin=[]  SumDenOutMax=[]  SumNumOutMin=[]  SumNumOutMax=[]  ReciprocalOutMin=[]  ReciprocalOutMax=[]  DivideOutMin=[]  DivideOutMax=[]  TunerSelectOption=Transfer Function Based (PID Tuner App)
  cfblk9 : Delay  DelayLengthSource=Input port
      settings: InputPortMap=u0,p1
  cyemi_{460..463,478..479,488..497} (16 alike) : DataTypeConversion  OutDataTypeStr=double
  cfblk2 : Outport
  cfblk14 : Outport  Port=2
  cfblk15 : Outport  Port=3
  wires:
  cfblk10/1 -> cfblk14/1, cyemi_492/1
  cfblk6/1 -> cfblk15/1, cyemi_488/1
  cfblk8/1 -> cfblk2/1, cyemi_461/1, cyemi_490/1
  cfblk11/1 -> cfblk16/Action
  cfblk11/2 -> cfblk17/Action
  cyemi_460/1 -> cfblk10/1
  cfblk13/1 -> cyemi_460/1
  cyemi_461/1 -> cfblk10/2
  cyemi_462/1 -> cfblk11/1
  cfblk12/1 -> cyemi_462/1
  cyemi_463/1 -> cfblk16/1(cfblk1)
  cfblk17/2(cfblk10) -> cyemi_463/1
  cyemi_478/1 -> cfblk17/1(cfblk1)
  cfblk5/1 -> cyemi_478/1
  cyemi_479/1 -> cfblk17/2(cfblk9)
  cfblk18/1 -> cyemi_479/1
  cyemi_488/1 -> cfblk18/1
  cyemi_489/1 -> cfblk3/1
  cfblk9/1 -> cyemi_489/1
  cyemi_490/1 -> cfblk4/1
  cyemi_491/1 -> cfblk5/1
  cfblk4/1 -> cyemi_491/1
  cyemi_492/1 -> cfblk5/2
  cyemi_493/1 -> cfblk6/1
  cfblk3/1 -> cyemi_493/1
  cyemi_494/1 -> cfblk7/1
  cfblk1/1 -> cyemi_494/1
  cyemi_495/1 -> cfblk8/1
  cfblk7/1 -> cyemi_495/1
  cyemi_496/1 -> cfblk9/1
  cfblk16/1(cfblk2) -> cyemi_496/1
  cyemi_497/1 -> cfblk9/2
  cfblk17/1(cfblk2) -> cyemi_497/1

== system equivalent/cfblk300 ==
  cfblk1 : Inport
  cfblk12 : Inport  Port=2
  Action Port : ActionPort  ActionType=else
  cfblk{7,10,17..18} (4 alike) : Delay
  cfblk11 : DiscreteIntegrator  SampleTime=-1  ICPrevOutput=DiscIntNeverNeededParam  ICPrevScaledInput=DiscIntNeverNeededParam
  cfblk3 : DiscreteFilter
  cfblk4 : simulink/Discrete/Tapped Delay  vinit=0.0  samptime=-1  NumDelays=1  DelayOrder=Oldest  includeCurrent=off
  cfblk5 : simulink/Continuous/PID Controller (2DOF)  Controller=PID  TimeDomain=Discrete-time  SampleTime=-1  IntegratorMethod=Forward Euler  FilterMethod=Forward Euler  Form=Parallel  UseFilter=on  ControllerParametersSource=internal  P=1  I=1  D=0  N=100  b=1  c=1  InitialConditionSource=internal  InitialConditionForIntegrator=0  InitialConditionForFilter=0  ExternalReset=none  LimitOutput=off  UpperSaturationLimit=inf  LowerSaturationLimit=-inf  LinearizeAsGain=off  AntiWindupMode=none  Kb=1  TrackingMode=off  Kt=1  PParamMin=[]  PParamMax=[]  IParamMin=[]  IParamMax=[]  DParamMin=[]  DParamMax=[]  NParamMin=[]  NParamMax=[]  bParamMin=[]  bParamMax=[]  cParamMin=[]  cParamMax=[]  KbParamMin=[]  KbParamMax=[]  KtParamMin=[]  KtParamMax=[]  POutMin=[]  POutMax=[]  IOutMin=[]  IOutMax=[]  DOutMin=[]  DOutMax=[]  NOutMin=[]  NOutMax=[]  bOutMin=[]  bOutMax=[]  cOutMin=[]  cOutMax=[]  KbOutMin=[]  KbOutMax=[]  KtOutMin=[]  KtOutMax=[]  IntegratorOutMin=[]  IntegratorOutMax=[]  FilterOutMin=[]  FilterOutMax=[]  SumOutMin=[]  SumOutMax=[]  Sum1OutMin=[]  Sum1OutMax=[]  Sum2OutMin=[]  Sum2OutMax=[]  Sum3OutMin=[]  Sum3OutMax=[]  SumI1OutMin=[]  SumI1OutMax=[]  SumI2OutMin=[]  SumI2OutMax=[]  SumI3OutMin=[]  SumI3OutMax=[]  SumDOutMin=[]  SumDOutMax=[]  SaturationOutMin=[]  SaturationOutMax=[]  IntegratorContinuousStateAttributes=''  IntegratorStateMustResolveToSignalObject=off  IntegratorRTWStateStorageClass=Auto  FilterContinuousStateAttributes=''  FilterStateMustResolveToSignalObject=off  FilterRTWStateStorageClass=Auto  DifferentiatorICPrevScaledInput=0  DifferentiatorOutMin=[]  DifferentiatorOutMax=[]  FilterDiffOutCoefMin=[]  FilterDiffOutCoefMax=[]  SumDenOutMin=[]  SumDenOutMax=[]  SumNumOutMin=[]  SumNumOutMax=[]  ReciprocalOutMin=[]  ReciprocalOutMax=[]  DivideOutMin=[]  DivideOutMax=[]  TunerSelectOption=Transfer Function Based (PID Tuner App)
  cfblk6 : Delay  DelayLengthSource=Input port
      settings: InputPortMap=u0,p1
  cfblk8 : DiscreteTransferFcn
  cfblk9 : Delay  DelayLengthSource=Input port
      settings: InputPortMap=u0,p1
  cyemi_{503..516} (14 alike) : DataTypeConversion  OutDataTypeStr=double
  cfblk2 : Outport
  cfblk13 : Outport  Port=2
  cfblk14 : Outport  Port=3
  cfblk15 : Outport  Port=4
  cfblk16 : Outport  Port=5
  wires:
  cfblk1/1 -> cyemi_508/1, cyemi_516/1
  cfblk12/1 -> cfblk14/1
  cfblk10/1 -> cfblk15/1, cyemi_512/1
  cfblk6/1 -> cyemi_510/1, cyemi_514/1
  cfblk11/1 -> cfblk13/1
  cfblk7/1 -> cyemi_504/1, cyemi_506/1
  cfblk5/1 -> cfblk2/1, cyemi_513/1, cyemi_515/1
  cfblk9/1 -> cfblk16/1
  cyemi_503/1 -> cfblk10/1
  cfblk3/1 -> cyemi_503/1
  cyemi_504/1 -> cfblk11/1
  cyemi_505/1 -> cfblk17/1
  cfblk8/1 -> cyemi_505/1
  cyemi_506/1 -> cfblk18/1
  cyemi_507/1 -> cfblk3/1
  cfblk4/1 -> cyemi_507/1
  cyemi_508/1 -> cfblk4/1
  cyemi_509/1 -> cfblk5/1
  cfblk18/1 -> cyemi_509/1
  cyemi_510/1 -> cfblk5/2
  cyemi_511/1 -> cfblk6/1
  cfblk17/1 -> cyemi_511/1
  cyemi_512/1 -> cfblk6/2
  cyemi_513/1 -> cfblk7/1
  cyemi_514/1 -> cfblk8/1
  cyemi_515/1 -> cfblk9/1
  cyemi_516/1 -> cfblk9/2

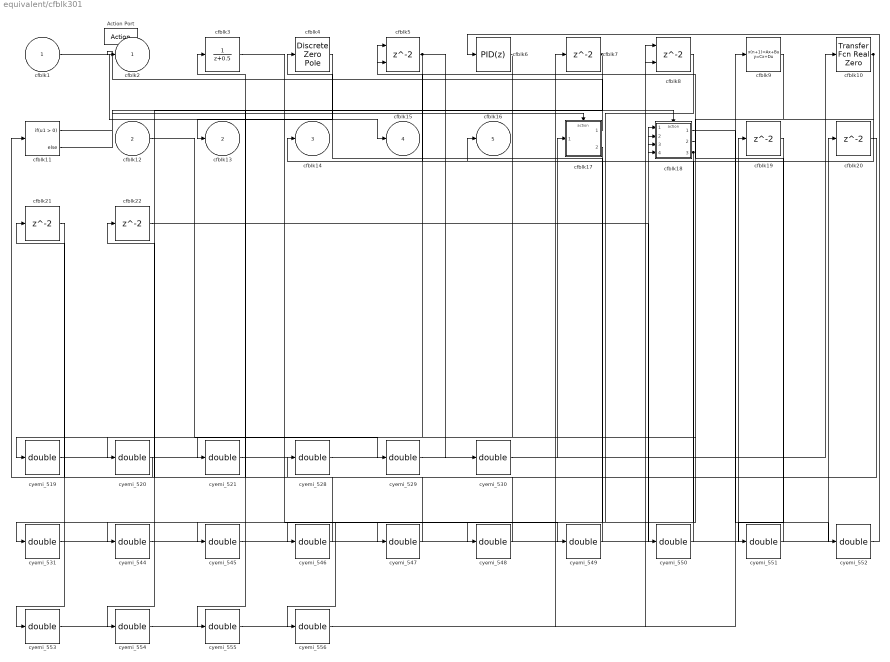
== system equivalent/cfblk301 ==
  cfblk1 : Inport
  cfblk12 : Inport  Port=2
  Action Port : ActionPort  ActionType=then
  cfblk10 : simulink/Discrete/Transfer Fcn Real Zero  ZeroZ=0.75  ICPrevInput=0.0  DoSatur=off
      settings: SourceProductName=Simulink  SourceProductBaseCode=SL
  cfblk11 : If  SampleTime=1
  cfblk17 : Subsystem  TreatAsAtomicUnit=on
  cfblk18 : Subsystem  TreatAsAtomicUnit=on
  cfblk{7,19..22} (5 alike) : Delay
  cfblk3 : DiscreteTransferFcn
  cfblk4 : DiscreteZeroPole  Poles=[0 0.5]  Gain=1  SampleTime=-1
  cfblk5 : Delay  ShowEnablePort=on
      settings: InputPortMap=u0,e6
  cfblk6 : simulink/Continuous/PID Controller  Controller=PID  TimeDomain=Discrete-time  SampleTime=-1  IntegratorMethod=Forward Euler  FilterMethod=Forward Euler  Form=Parallel  UseFilter=on  ControllerParametersSource=internal  P=1  I=1  D=0  N=100  InitialConditionSource=internal  InitialConditionForIntegrator=0  InitialConditionForFilter=0  ExternalReset=none  LimitOutput=off  UpperSaturationLimit=inf  LowerSaturationLimit=-inf  LinearizeAsGain=off  AntiWindupMode=none  Kb=1  TrackingMode=off  Kt=1  PParamMin=[]  PParamMax=[]  IParamMin=[]  IParamMax=[]  DParamMin=[]  DParamMax=[]  NParamMin=[]  NParamMax=[]  KbParamMin=[]  KbParamMax=[]  KtParamMin=[]  KtParamMax=[]  POutMin=[]  POutMax=[]  IOutMin=[]  IOutMax=[]  DOutMin=[]  DOutMax=[]  NOutMin=[]  NOutMax=[]  KbOutMin=[]  KbOutMax=[]  KtOutMin=[]  KtOutMax=[]  IntegratorOutMin=[]  IntegratorOutMax=[]  FilterOutMin=[]  FilterOutMax=[]  SumOutMin=[]  SumOutMax=[]  SumI1OutMin=[]  SumI1OutMax=[]  SumI2OutMin=[]  SumI2OutMax=[]  SumI3OutMin=[]  SumI3OutMax=[]  SumDOutMin=[]  SumDOutMax=[]  SaturationOutMin=[]  SaturationOutMax=[]  IntegratorContinuousStateAttributes=''  IntegratorStateMustResolveToSignalObject=off  IntegratorRTWStateStorageClass=Auto  FilterContinuousStateAttributes=''  FilterStateMustResolveToSignalObject=off  FilterRTWStateStorageClass=Auto  DifferentiatorICPrevScaledInput=0  DifferentiatorOutMin=[]  DifferentiatorOutMax=[]  FilterDiffOutCoefMin=[]  FilterDiffOutCoefMax=[]  SumDenOutMin=[]  SumDenOutMax=[]  SumNumOutMin=[]  SumNumOutMax=[]  ReciprocalOutMin=[]  ReciprocalOutMax=[]  DivideOutMin=[]  DivideOutMax=[]  TunerSelectOption=Transfer Function Based (PID Tuner App)
  cfblk8 : Delay  ShowEnablePort=on
      settings: InputPortMap=u0,e6
  cfblk9 : DiscreteStateSpace  SampleTime=-1
  cyemi_{519..521,528..531,544..556} (20 alike) : DataTypeConversion  OutDataTypeStr=double
  cfblk2 : Outport
  cfblk13 : Outport  Port=2
  cfblk14 : Outport  Port=3
  cfblk15 : Outport  Port=4
  cfblk16 : Outport  Port=5
  wires:
  cfblk1/1 -> cfblk15/1
  cfblk10/1 -> cfblk14/1, cyemi_548/1
  cfblk17/1(cfblk2) -> cfblk2/1
  cfblk5/1 -> cyemi_519/1, cyemi_520/1, cyemi_530/1
  cfblk18/3(cfblk16) -> cfblk16/1, cyemi_553/1, cyemi_556/1
  cfblk4/1 -> cfblk13/1
  cfblk11/1 -> cfblk17/Action
  cfblk11/2 -> cfblk18/Action
  cyemi_519/1 -> cfblk10/1
  cyemi_520/1 -> cfblk11/1
  cyemi_521/1 -> cfblk17/1(cfblk1)
  cfblk18/2(cfblk15) -> cyemi_521/1
  cyemi_528/1 -> cfblk18/1(cfblk1)
  cfblk20/1 -> cyemi_528/1
  cyemi_529/1 -> cfblk18/2(cfblk12)
  cfblk12/1 -> cyemi_529/1
  cyemi_530/1 -> cfblk18/3(cfblk13)
  cyemi_531/1 -> cfblk18/4(cfblk14)
  cfblk21/1 -> cyemi_531/1
  cyemi_544/1 -> cfblk19/1
  cfblk6/1 -> cyemi_544/1
  cyemi_545/1 -> cfblk20/1
  cfblk17/2(cfblk8) -> cyemi_545/1
  cyemi_546/1 -> cfblk21/1
  cfblk8/1 -> cyemi_546/1
  cyemi_547/1 -> cfblk22/1
  cfblk9/1 -> cyemi_547/1
  cyemi_548/1 -> cfblk3/1
  cyemi_549/1 -> cfblk4/1
  cfblk3/1 -> cyemi_549/1
  cyemi_550/1 -> cfblk5/1
  cfblk22/1 -> cyemi_550/1
  cyemi_551/1 -> cfblk5/2
  cfblk19/1 -> cyemi_551/1
  cyemi_552/1 -> cfblk6/1
  cfblk18/1(cfblk2) -> cyemi_552/1
  cyemi_553/1 -> cfblk7/1
  cyemi_554/1 -> cfblk8/1
  cfblk7/1 -> cyemi_554/1, cyemi_555/1
  cyemi_555/1 -> cfblk8/2
  cyemi_556/1 -> cfblk9/1

== system equivalent/cfblk302 ==
  cfblk1 : Inport
  Action Port : ActionPort  ActionType=else
  cfblk{10,17..19} (4 alike) : Delay
  cfblk11 : UnitDelay  SampleTime=-1
  cfblk12 : If  SampleTime=1
  cfblk15 : Subsystem  TreatAsAtomicUnit=on
  cfblk16 : Subsystem  TreatAsAtomicUnit=on
  cfblk20 : DataTypeConversion  OutDataTypeStr=double
  cfblk3 : simulink/Continuous/PID Controller (2DOF)  Controller=PID  TimeDomain=Discrete-time  SampleTime=-1  IntegratorMethod=Forward Euler  FilterMethod=Forward Euler  Form=Parallel  UseFilter=on  ControllerParametersSource=internal  P=1  I=1  D=0  N=100  b=1  c=1  InitialConditionSource=internal  InitialConditionForIntegrator=0  InitialConditionForFilter=0  ExternalReset=none  LimitOutput=off  UpperSaturationLimit=inf  LowerSaturationLimit=-inf  LinearizeAsGain=off  AntiWindupMode=none  Kb=1  TrackingMode=off  Kt=1  PParamMin=[]  PParamMax=[]  IParamMin=[]  IParamMax=[]  DParamMin=[]  DParamMax=[]  NParamMin=[]  NParamMax=[]  bParamMin=[]  bParamMax=[]  cParamMin=[]  cParamMax=[]  KbParamMin=[]  KbParamMax=[]  KtParamMin=[]  KtParamMax=[]  POutMin=[]  POutMax=[]  IOutMin=[]  IOutMax=[]  DOutMin=[]  DOutMax=[]  NOutMin=[]  NOutMax=[]  bOutMin=[]  bOutMax=[]  cOutMin=[]  cOutMax=[]  KbOutMin=[]  KbOutMax=[]  KtOutMin=[]  KtOutMax=[]  IntegratorOutMin=[]  IntegratorOutMax=[]  FilterOutMin=[]  FilterOutMax=[]  SumOutMin=[]  SumOutMax=[]  Sum1OutMin=[]  Sum1OutMax=[]  Sum2OutMin=[]  Sum2OutMax=[]  Sum3OutMin=[]  Sum3OutMax=[]  SumI1OutMin=[]  SumI1OutMax=[]  SumI2OutMin=[]  SumI2OutMax=[]  SumI3OutMin=[]  SumI3OutMax=[]  SumDOutMin=[]  SumDOutMax=[]  SaturationOutMin=[]  SaturationOutMax=[]  IntegratorContinuousStateAttributes=''  IntegratorStateMustResolveToSignalObject=off  IntegratorRTWStateStorageClass=Auto  FilterContinuousStateAttributes=''  FilterStateMustResolveToSignalObject=off  FilterRTWStateStorageClass=Auto  DifferentiatorICPrevScaledInput=0  DifferentiatorOutMin=[]  DifferentiatorOutMax=[]  FilterDiffOutCoefMin=[]  FilterDiffOutCoefMax=[]  SumDenOutMin=[]  SumDenOutMax=[]  SumNumOutMin=[]  SumNumOutMax=[]  ReciprocalOutMin=[]  ReciprocalOutMax=[]  DivideOutMin=[]  DivideOutMax=[]  TunerSelectOption=Transfer Function Based (PID Tuner App)
  cfblk4 : simulink/Discrete/Transfer Fcn Real Zero  ZeroZ=0.75  ICPrevInput=0.0  DoSatur=off
      settings: SourceProductName=Simulink  SourceProductBaseCode=SL
  cfblk5 : DiscreteIntegrator  SampleTime=-1  ICPrevOutput=DiscIntNeverNeededParam  ICPrevScaledInput=DiscIntNeverNeededParam
  cfblk6 : DiscreteIntegrator  SampleTime=-1  ICPrevOutput=DiscIntNeverNeededParam  ICPrevScaledInput=DiscIntNeverNeededParam
  cfblk7 : DiscreteFir
  cfblk8 : simulink/Discrete/Transfer Fcn Real Zero  ZeroZ=0.75  ICPrevInput=0.0  DoSatur=off
      settings: SourceProductName=Simulink  SourceProductBaseCode=SL
  cfblk9 : simulink/Discrete/Tapped Delay  vinit=0.0  samptime=-1  NumDelays=1  DelayOrder=Oldest  includeCurrent=off
  cyemi_558 : DataTypeConversion  OutDataTypeStr=uint32
  cyemi_559 : DataTypeConversion  OutDataTypeStr=uint32
  cyemi_{560..562,568..570,583..594} (18 alike) : DataTypeConversion  OutDataTypeStr=double
  cfblk2 : Outport
  cfblk13 : Outport  Port=2
  cfblk14 : Outport  Port=3
  wires:
  cfblk6/1 -> cfblk14/1
  cfblk16/1(cfblk2) -> cfblk2/1
  cfblk11/1 -> cfblk13/1
  cfblk8/1 -> cyemi_584/1, cyemi_591/1
  cfblk9/1 -> cyemi_560/1, cyemi_592/1
  cfblk12/1 -> cfblk15/Action
  cfblk12/2 -> cfblk16/Action
  cfblk20/1 -> cyemi_594/1, cyemi_590/1
  cyemi_558/1 -> cfblk10/1
  cfblk5/1 -> cyemi_558/1
  cyemi_559/1 -> cfblk11/1
  cfblk10/1 -> cyemi_559/1
  cyemi_560/1 -> cfblk12/1
  cyemi_561/1 -> cfblk15/1(cfblk1)
  cfblk19/1 -> cyemi_561/1
  cyemi_562/1 -> cfblk15/2(cfblk6)
  cfblk7/1 -> cyemi_562/1
  cyemi_568/1 -> cfblk16/1(cfblk1)
  cfblk17/1 -> cyemi_568/1
  cyemi_569/1 -> cfblk16/2(cfblk10)
  cfblk15/2(cfblk7) -> cyemi_569/1
  cyemi_570/1 -> cfblk16/3(cfblk11)
  cfblk18/1 -> cyemi_570/1
  cyemi_583/1 -> cfblk17/1
  cfblk4/1 -> cyemi_583/1
  cyemi_584/1 -> cfblk18/1
  cyemi_585/1 -> cfblk19/1
  cfblk3/1 -> cyemi_585/1
  cyemi_586/1 -> cfblk20/1
  cfblk1/1 -> cyemi_586/1
  cyemi_587/1 -> cfblk3/1
  cfblk16/3(cfblk13) -> cyemi_587/1
  cyemi_588/1 -> cfblk3/2
  cfblk16/4(cfblk14) -> cyemi_588/1
  cyemi_589/1 -> cfblk4/1
  cfblk15/1(cfblk2) -> cyemi_589/1
  cyemi_590/1 -> cfblk5/1
  cyemi_591/1 -> cfblk6/1
  cyemi_592/1 -> cfblk7/1
  cyemi_593/1 -> cfblk8/1
  cfblk16/2(cfblk12) -> cyemi_593/1
  cyemi_594/1 -> cfblk9/1
